simulink model "motordc_simu"  (R2025a)
settings: Solver=VariableStepAuto  StartTime=0.0  StopTime=10.0  RelTol=1e-3
PreLoadFcn:
  | Ra=2;
  | Kt=0.01;
  | B=0.0012;
  | La=0.023;
  | Ke=0.01;
  | J=0.001;
  | Va=32;
  | Tl=0;
settings Model: Creator=Chris  LastModifiedBy=Chris

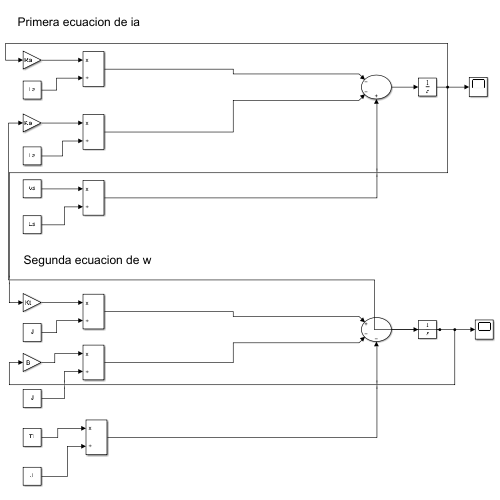
[thumbnail: Simulink's stored preview of the top-level diagram]
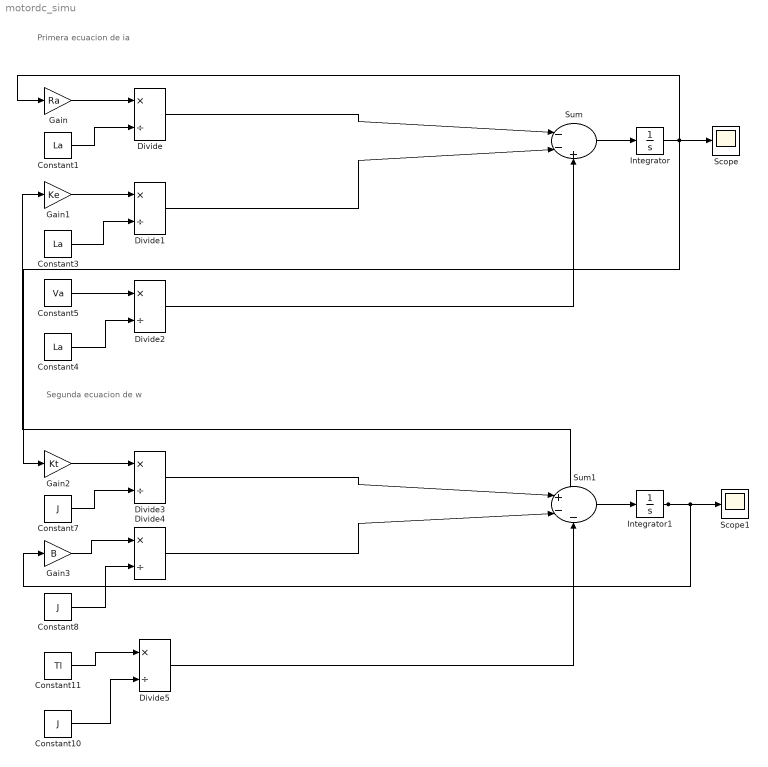
== system motordc_simu ==
  note: Primera ecuacion de ia
  note: Segunda ecuacion de w
  Constant1 : Constant  Value=La
  Constant10 : Constant  Value=J
  Constant11 : Constant  Value=Tl
  Constant3 : Constant  Value=La
  Constant4 : Constant  Value=La
  Constant5 : Constant  Value=Va
  Constant7 : Constant  Value=J
  Constant8 : Constant  Value=J
  Divide{,1..5} (6 alike) : Product  Inputs=*/
  Gain : Gain  Gain=Ra
  Gain1 : Gain  Gain=Ke
  Gain2 : Gain  Gain=Kt
  Gain3 : Gain  Gain=B
  Integrator : Integrator
  Integrator1 : Integrator
  Scope : Scope
      settings: ActiveDisplayYMinimum=-1.9926432992408414  ActiveDisplayYMaximum=17.933789693167576
  Scope1 : Scope
      settings: ActiveDisplayYMinimum=-16.00014672578622  ActiveDisplayYMaximum=144.00132053207602
  Sum : Sum  Inputs=|--+
  Sum1 : Sum  Inputs=|+--
  wires:
  Integrator/1 -> Gain/1, Gain2/1, Scope/1
  Gain/1 -> Divide/1
  Constant1/1 -> Divide/2
  Divide/1 -> Sum/1
  Gain1/1 -> Divide1/1
  Constant3/1 -> Divide1/2
  Divide1/1 -> Sum/2
  Constant4/1 -> Divide2/2
  Constant5/1 -> Divide2/1
  Divide2/1 -> Sum/3
  Sum/1 -> Integrator/1
  Constant7/1 -> Divide3/2
  Divide3/1 -> Sum1/1
  Gain2/1 -> Divide3/1
  Constant8/1 -> Divide4/2
  Gain3/1 -> Divide4/1
  Integrator1/1 -> Gain3/1, Scope1/1, Gain1/1
  Divide4/1 -> Sum1/2
  Constant10/1 -> Divide5/2
  Constant11/1 -> Divide5/1
  Divide5/1 -> Sum1/3
  Sum1/1 -> Integrator1/1
